simulink model "simuelectrico"  (R2024b)
settings: Solver=VariableStepAuto  StartTime=0.0  StopTime=0.01  RelTol=1e-3
InitFcn:
  | l=0.002;
  | r=10;
  | c=10*10^-6;
  | u=32;
  | d=0.4;
  | f_pwm = 100000;
settings Model: Creator=Fernando  LastModifiedBy=Fernando

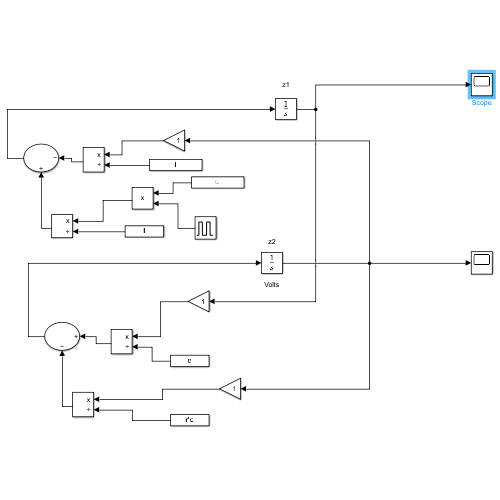
[thumbnail: Simulink's stored preview of the top-level diagram]
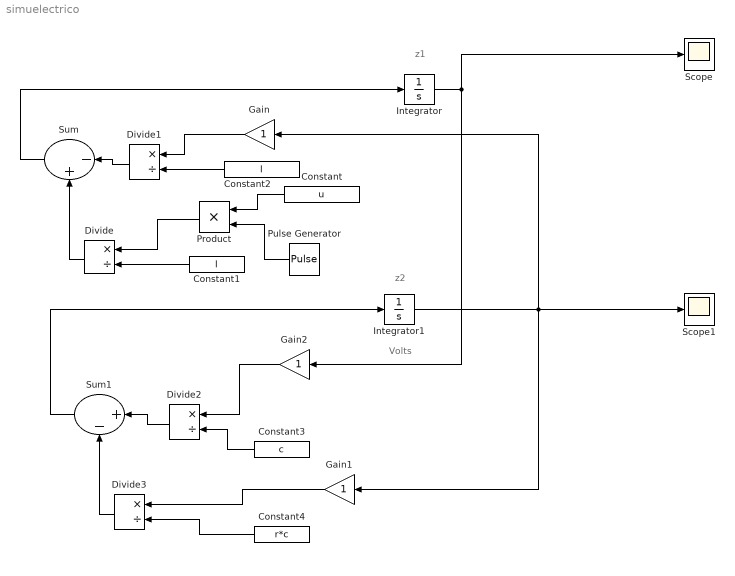
== system simuelectrico ==
  note: Volts
  note: z1
  note: z2
  Constant : Constant  Value=u
  Constant1 : Constant  Value=l
  Constant2 : Constant  Value=l
  Constant3 : Constant  Value=c
  Constant4 : Constant  Value=r*c
  Divide{,1..3} (4 alike) : Product  Inputs=*/
  Gain : Gain
  Gain1 : Gain
  Gain2 : Gain
  Integrator : Integrator
  Integrator1 : Integrator
  Product : Product
  Pulse Generator : DiscretePulseGenerator  PulseType=Time based  Period=1/100e3  PulseWidth=40
  Scope : Scope
  Scope1 : Scope
  Sum : Sum  Inputs=|-+
  Sum1 : Sum  Inputs=|+-
  wires:
  Integrator/1 -> Gain2/1, Scope/1
  Integrator1/1 -> Gain1/1, Gain/1, Scope1/1
  Sum/1 -> Integrator/1
  Sum1/1 -> Integrator1/1
  Divide/1 -> Sum/2
  Constant1/1 -> Divide/2
  Divide1/1 -> Sum/1
  Divide2/1 -> Sum1/1
  Divide3/1 -> Sum1/2
  Product/1 -> Divide/1
  Constant/1 -> Product/1
  Pulse Generator/1 -> Product/2
  Constant4/1 -> Divide3/2
  Gain/1 -> Divide1/1
  Constant2/1 -> Divide1/2
  Gain1/1 -> Divide3/1
  Constant3/1 -> Divide2/2
  Gain2/1 -> Divide2/1
